simulink model "StateObserver"  (R2021b)
settings: Solver=VariableStepAuto  StartTime=0.0  StopTime=30.0  RelTol=1e-3
values from neighbouring files (symbols this model uses):
  A = [0 0  1  0 ... (first row only)    [CartPend.m]    (also in ExB.m = Gz.a; Input of ExD.mat = [1 0 0 0 1.98988607898e-05 0.999628951737 0.00784288446048 -)
  B = PWMgain*[0;0;b1;b2]    [CartPend.m]    (also in ExB.m = Gz.b; Input of ExD.mat = [0.000160700219307 -0.000418368578462 0.063341441113 -0.1648)
  C = [1 0 0 0;0 1 0 0]    [CartPend.m]    (also in ExB.m = Gz.c; Input of ExD.mat = [1  0  0  0; 0  1  0  0])
  D = [0;0]    [CartPend.m]    (also in ExB.m = Gz.d; Input of ExD.mat = [0 0])
  L = 0.6    [CartPend.m]    (also in ExB.m = place(A', C', Po)'; Input of ExD.mat = [0.910764301089  -0.150385746241; 0.338160576948  0.95137784; NLpendulum.m)
libraries: simulink x1
settings Model: Creator=westwick  LastModifiedBy=Andrey
settings SolverCC: AlgebraicLoopSolver=TrustRegion
settings DebuggingCC: SFMachineParentedDataDiag=warning
settings SFSimCC: CustomCodeUndefinedFunction=UseInterfaceOnly

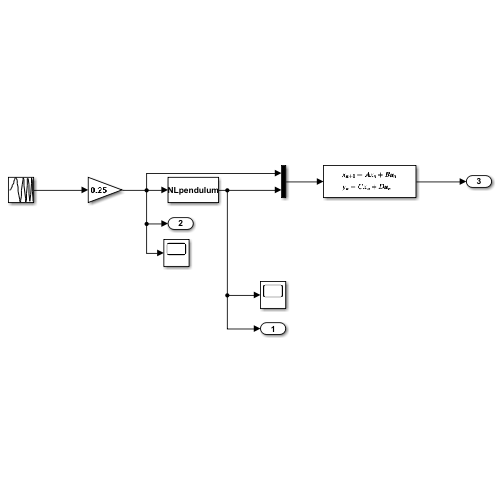
[thumbnail: Simulink's stored preview of the top-level diagram]
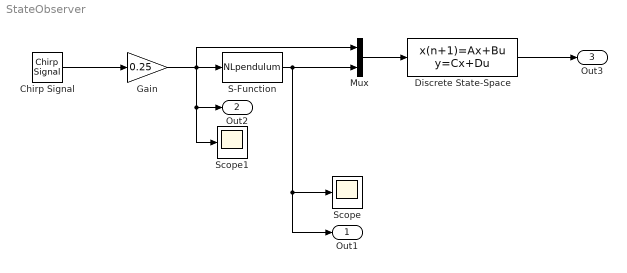
== system StateObserver ==
  Chirp Signal : simulink/Sources/Chirp Signal  f1=0.2  T=30  f2=2
  Discrete State-Space : DiscreteStateSpace  A=A-(L*C)  B=[B-L*D , L]  C=eye(4)  D=zeros(4,3)  SampleTime=1/200
  Gain : Gain  Gain=0.25
  Mux : Mux  Inputs=2
  S-Function : S-Function  FunctionName=NLpendulum  SFunctionDeploymentMode=off  EnableBusSupport=off
  Scope : Scope
  Scope1 : Scope
  Out1 : Outport  VectorParamsAs1DForOutWhenUnconnected=off
  Out2 : Outport  Port=2  VectorParamsAs1DForOutWhenUnconnected=off
  Out3 : Outport  Port=3
  wires:
  Gain/1 -> Mux/1, Out2/1, Scope1/1, S-Function/1
  Chirp Signal/1 -> Gain/1
  S-Function/1 -> Mux/2, Out1/1, Scope/1
  Mux/1 -> Discrete State-Space/1
  Discrete State-Space/1 -> Out3/1
